simulink model "es2_3"  (R2022b)
settings: Solver=FixedStepDiscrete  StartTime=0.0  StopTime=30  RelTol=1e-3
values from neighbouring files (symbols this model uses):
  b = fir1(filterOrder, [low, high], 'bandpass')    [data_matrix.m]
  b_lp = fir1(filterOrder, low_cutoff, 'low')    [data_matrix.m]
libraries: vrlib x2
settings Model: Creator=simon  LastModifiedBy=franc
settings SolverCC: AlgebraicLoopSolver=TrustRegion  AutoInsertRateTranBlk=on
settings DataIOCC: LimitDataPoints=on  SaveOutput=off  SignalLogging=off  DSMLogging=off  SaveTime=off
settings OptimizationCC: ReuseModelBlockBuffer=on  LifeSpan=inf
settings DebuggingCC: AlgebraicLoopMsg=error  SingleTaskRateTransMsg=error  UnconnectedInputMsg=warning  UnconnectedOutputMsg=warning  UnconnectedLineMsg=warning  AllowSymbolicDim=off  SFUnexpectedBacktrackingDiag=warning  SFNoUnconditionalDefaultTransitionDiag=warning  SFExecutionAtInitializationDiag=none  ArithmeticOperatorsInVariantConditions=warning
settings ModelReferenceCC: EnableRefExpFcnMdlSchedulingChecks=on
settings SFSimCC: SimUseLocalCustomCode=off  CustomCodeUndefinedFunction=UseInterfaceOnly
settings RTWCC: RTWUseLocalCustomCode=off
settings CodeAppCC: StateflowObjectComments=on
settings GRTTargetCC: TargetLangStandard=C89/C90 (ANSI)

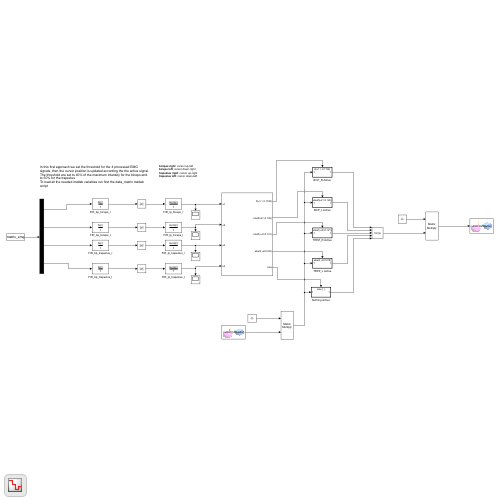
[thumbnail: Simulink's stored preview of the top-level diagram]
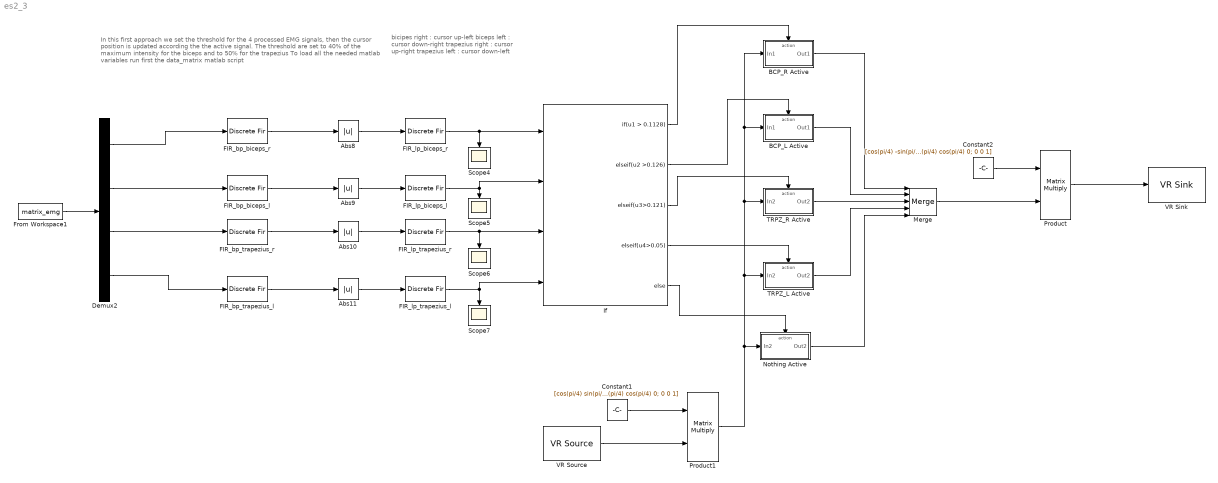
== system es2_3 ==
  note: bicipes right : cursor up-left
      | biceps left : cursor down-right
      | trapezius right : cursor up-right
      | trapezius left : cursor down-left
  note: In this first approach we set the threshold for the 4 processed EMG signals, then the cursor position is updated according the the active signal. The threshold are set to 40% of the maximum intensity for the biceps and to 50% for the trapezius
      | To load all the needed matlab variables run first the data_matrix matlab script
  Abs{8..11} (4 alike) : Abs  SaturateOnIntegerOverflow=off
  BCP_L Active : Subsystem  TreatAsAtomicUnit=on
  BCP_R Active : Subsystem  TreatAsAtomicUnit=on
  Constant1 : Constant  Value=[cos(pi/4) sin(pi/4) 0; -sin(pi/4) cos(pi/4) 0; 0 0 1]  SampleTime=1/1000
  Constant2 : Constant  Value=[cos(pi/4) -sin(pi/4) 0; sin(pi/4) cos(pi/4) 0; 0 0 1]  SampleTime=1/1000
  Demux2 : Demux
  FIR_bp_biceps_l : DiscreteFir  Coefficients=b
  FIR_bp_biceps_r : DiscreteFir  Coefficients=b
  FIR_bp_trapezius_l : DiscreteFir  Coefficients=b
  FIR_bp_trapezius_r : DiscreteFir  Coefficients=b
  FIR_lp_biceps_l : DiscreteFir  Coefficients=b_lp
  FIR_lp_biceps_r : DiscreteFir  Coefficients=b_lp
  FIR_lp_trapezius_l : DiscreteFir  Coefficients=b_lp
  FIR_lp_trapezius_r : DiscreteFir  Coefficients=b_lp
  From Workspace1 : FromWorkspace  VariableName=matrix_emg  SampleTime=1/1000
  If : If  NumInputs=4  IfExpression=u1 > 0.1128  ElseIfExpressions=u2 >0.126, u3>0.121, u4>0.05
  Merge : Merge  Inputs=5
  Nothing Active : Subsystem  TreatAsAtomicUnit=on
  Product : Product  Multiplication=Matrix(*)
  Product1 : Product  Multiplication=Matrix(*)
  Scope{4..7} (4 alike) : Scope
  TRPZ_L Active : Subsystem  TreatAsAtomicUnit=on
  TRPZ_R Active : Subsystem  TreatAsAtomicUnit=on
  VR Sink : vrlib/VR Sink  InstantiateOnLoad=on  SampleTime=1/1000  ViewEnable=on  RemoteChange=off  RemoteView=off  FieldsWritten=cursor.translation.3.1.1.double  WorldFileName=8_palline_color.wrl  AutoView=off  VideoDimensions=[]  AllowVariableSize=off  FigureProperties=[]
  VR Source : vrlib/VR Source  InstantiateOnLoad=on  SampleTime=1/1000  ViewEnable=on  RemoteChange=off  RemoteView=off  FieldsRead=cursor.translation.1.3.1.double  WorldFileName=8_palline_color.wrl  AutoView=off  VideoDimensions=[]  AllowVariableSize=off  FigureProperties=[]
  wires:
  Constant2/1 -> Product/1
  Product/1 -> VR Sink/1
  BCP_R Active/1(Out1) -> Merge/1
  FIR_bp_trapezius_l/1 -> Abs11/1
  Nothing Active/1(Out2) -> Merge/5
  TRPZ_R Active/1(Out2) -> Merge/3
  Abs10/1 -> FIR_lp_trapezius_r/1
  Demux2/4 -> FIR_bp_trapezius_l/1
  FIR_bp_biceps_l/1 -> Abs9/1
  Demux2/3 -> FIR_bp_trapezius_r/1
  BCP_L Active/1(Out1) -> Merge/2
  FIR_lp_biceps_r/1 -> Scope4/1, If/1
  FIR_bp_biceps_r/1 -> Abs8/1
  Merge/1 -> Product/2
  FIR_lp_trapezius_l/1 -> Scope7/1, If/4
  Demux2/2 -> FIR_bp_biceps_l/1
  FIR_lp_trapezius_r/1 -> Scope6/1, If/3
  Abs11/1 -> FIR_lp_trapezius_l/1
  TRPZ_L Active/1(Out2) -> Merge/4
  Abs8/1 -> FIR_lp_biceps_r/1
  If/1 -> BCP_R Active/Action
  If/4 -> TRPZ_L Active/Action
  If/5 -> Nothing Active/Action
  VR Source/1 -> Product1/2
  If/2 -> BCP_L Active/Action
  If/3 -> TRPZ_R Active/Action
  Demux2/1 -> FIR_bp_biceps_r/1
  Abs9/1 -> FIR_lp_biceps_l/1
  From Workspace1/1 -> Demux2/1
  FIR_lp_biceps_l/1 -> If/2, Scope5/1
  FIR_bp_trapezius_r/1 -> Abs10/1
  Constant1/1 -> Product1/1
  Product1/1 -> Nothing Active/1(In2), TRPZ_L Active/1(In2), TRPZ_R Active/1(In2), BCP_L Active/1(In1), BCP_R Active/1(In1)

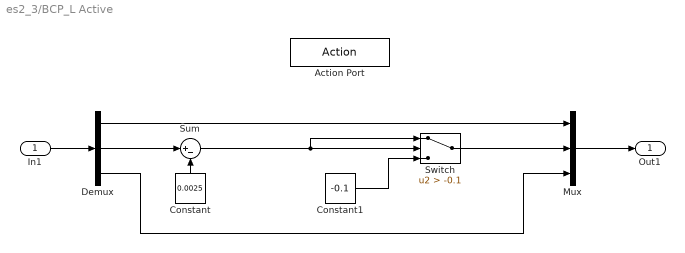
== system es2_3/BCP_L Active ==
  In1 : Inport
  Action Port : ActionPort  ActionPortLabel=elseif(u2 >0.126)
  Constant : Constant  Value=0.0025  SampleTime=1/1000
  Constant1 : Constant  Value=-0.1  SampleTime=1/1000
  Demux : Demux  Outputs=3
  Mux : Mux  Inputs=3
  Sum : Sum  Inputs=|+-  OutMin=[-0.1]  OutMax=[0]
  Switch : Switch  Criteria=u2 > Threshold  Threshold=-0.1  SaturateOnIntegerOverflow=off  InputSameDT=off
  Out1 : Outport
  wires:
  Demux/3 -> Mux/3
  In1/1 -> Demux/1
  Mux/1 -> Out1/1
  Constant/1 -> Sum/2
  Demux/1 -> Mux/1
  Demux/2 -> Sum/1
  Sum/1 -> Switch/1, Switch/2
  Switch/1 -> Mux/2
  Constant1/1 -> Switch/3

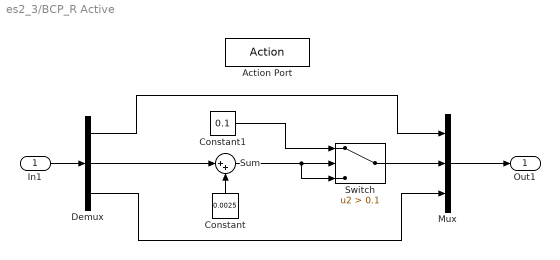
== system es2_3/BCP_R Active ==
  In1 : Inport
  Action Port : ActionPort  ActionPortLabel=if(u1 > 0.1128)
  Constant : Constant  Value=0.0025  SampleTime=1/1000
  Constant1 : Constant  Value=0.1  SampleTime=1/1000
  Demux : Demux  Outputs=3
  Mux : Mux  Inputs=3
  Sum : Sum  Inputs=|++  OutMin=[0]  OutMax=[0.1]
  Switch : Switch  Criteria=u2 > Threshold  Threshold=0.1  SaturateOnIntegerOverflow=off  InputSameDT=off
  Out1 : Outport
  wires:
  Constant/1 -> Sum/2
  In1/1 -> Demux/1
  Demux/2 -> Sum/1
  Mux/1 -> Out1/1
  Sum/1 -> Switch/3, Switch/2
  Demux/1 -> Mux/1
  Demux/3 -> Mux/3
  Constant1/1 -> Switch/1
  Switch/1 -> Mux/2

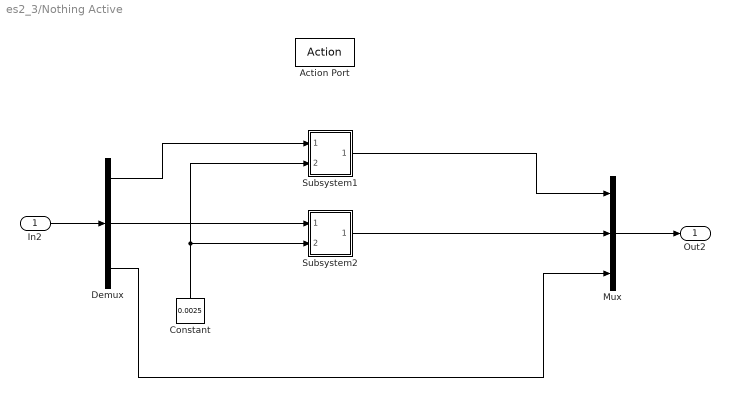
== system es2_3/Nothing Active ==
  In2 : Inport
  Action Port : ActionPort  ActionPortLabel=else
  Constant : Constant  Value=0.0025  SampleTime=1/1000
  Demux : Demux  Outputs=3
  Mux : Mux  Inputs=3
  Subsystem1 : Subsystem
  Subsystem2 : Subsystem
  Out2 : Outport
  wires:
  Mux/1 -> Out2/1
  Demux/3 -> Mux/3
  In2/1 -> Demux/1
  Constant/1 -> Subsystem2/2(In2), Subsystem1/2(In2)
  Subsystem2/1(Out1) -> Mux/2
  Demux/1 -> Subsystem1/1(In1)
  Subsystem1/1(Out1) -> Mux/1
  Demux/2 -> Subsystem2/1(In1)

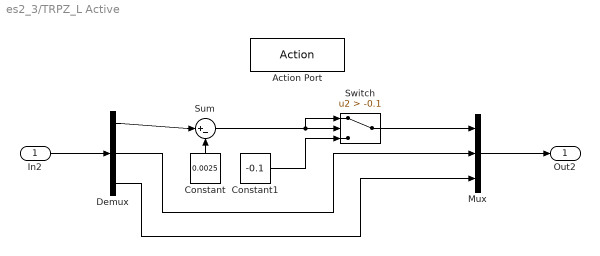
== system es2_3/TRPZ_L Active ==
  In2 : Inport
  Action Port : ActionPort  ActionPortLabel=elseif( u4>0.05)
  Constant : Constant  Value=0.0025  SampleTime=1/1000
  Constant1 : Constant  Value=-0.1  SampleTime=1/1000
  Demux : Demux  Outputs=3
  Mux : Mux  Inputs=3
  Sum : Sum  Inputs=|+-  OutMin=[-0.1]  OutMax=[0]
  Switch : Switch  Criteria=u2 > Threshold  Threshold=-0.1  SaturateOnIntegerOverflow=off  InputSameDT=off
  Out2 : Outport
  wires:
  Demux/1 -> Sum/1
  Constant/1 -> Sum/2
  Demux/2 -> Mux/2
  Mux/1 -> Out2/1
  Demux/3 -> Mux/3
  In2/1 -> Demux/1
  Constant1/1 -> Switch/3
  Switch/1 -> Mux/1
  Sum/1 -> Switch/1, Switch/2

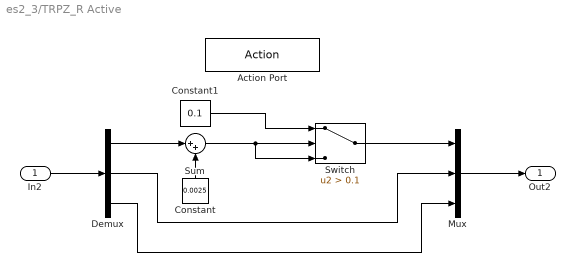
== system es2_3/TRPZ_R Active ==
  In2 : Inport
  Action Port : ActionPort  ActionPortLabel=elseif( u3>0.121)
  Constant : Constant  Value=0.0025  SampleTime=1/1000
  Constant1 : Constant  Value=0.1
  Demux : Demux  Outputs=3
  Mux : Mux  Inputs=3
  Sum : Sum  Inputs=|++  OutMin=[0]  OutMax=[0.1]
  Switch : Switch  Criteria=u2 > Threshold  Threshold=0.1  SaturateOnIntegerOverflow=off  InputSameDT=off
  Out2 : Outport
  wires:
  Demux/3 -> Mux/3
  In2/1 -> Demux/1
  Mux/1 -> Out2/1
  Constant/1 -> Sum/2
  Demux/1 -> Sum/1
  Demux/2 -> Mux/2
  Constant1/1 -> Switch/1
  Switch/1 -> Mux/1
  Sum/1 -> Switch/3, Switch/2

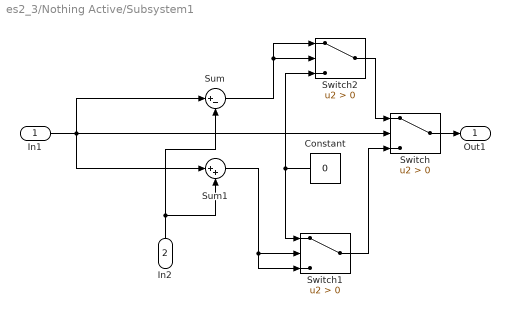
== system es2_3/Nothing Active/Subsystem1 ==
  In1 : Inport
  In2 : Inport  Port=2
  Constant : Constant  Value=0  SampleTime=1/1000
  Sum : Sum  Inputs=|+-
  Sum1 : Sum  Inputs=|++
  Switch : Switch  Criteria=u2 > Threshold  SaturateOnIntegerOverflow=off  InputSameDT=off
  Switch1 : Switch  Criteria=u2 > Threshold  SaturateOnIntegerOverflow=off  InputSameDT=off
  Switch2 : Switch  Criteria=u2 > Threshold  SaturateOnIntegerOverflow=off  InputSameDT=off
  Out1 : Outport
  wires:
  Switch/1 -> Out1/1
  Sum1/1 -> Switch1/2, Switch1/3
  In1/1 -> Switch/2, Sum/1, Sum1/1
  In2/1 -> Sum1/2, Sum/2
  Constant/1 -> Switch2/3, Switch1/1
  Switch1/1 -> Switch/3
  Switch2/1 -> Switch/1
  Sum/1 -> Switch2/2, Switch2/1

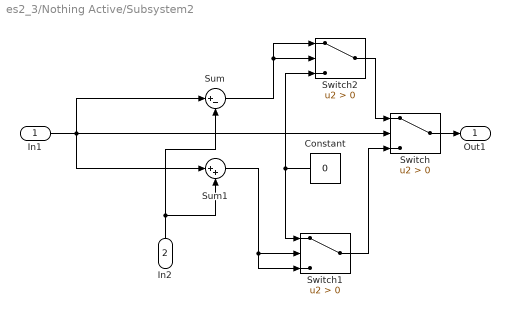
== system es2_3/Nothing Active/Subsystem2 ==
  In1 : Inport
  In2 : Inport  Port=2
  Constant : Constant  Value=0  SampleTime=1/1000
  Sum : Sum  Inputs=|+-
  Sum1 : Sum  Inputs=|++
  Switch : Switch  Criteria=u2 > Threshold  SaturateOnIntegerOverflow=off  InputSameDT=off
  Switch1 : Switch  Criteria=u2 > Threshold  SaturateOnIntegerOverflow=off  InputSameDT=off
  Switch2 : Switch  Criteria=u2 > Threshold  SaturateOnIntegerOverflow=off  InputSameDT=off
  Out1 : Outport
  wires:
  Switch/1 -> Out1/1
  Sum1/1 -> Switch1/2, Switch1/3
  In1/1 -> Switch/2, Sum/1, Sum1/1
  In2/1 -> Sum1/2, Sum/2
  Constant/1 -> Switch2/3, Switch1/1
  Switch1/1 -> Switch/3
  Switch2/1 -> Switch/1
  Sum/1 -> Switch2/2, Switch2/1
